simulink model "TinBotEliminator"  (Simulink 8.7)
settings: Solver=VariableStepAuto  StartTime=0.0  StopTime=10.0  RelTol=1e-3
settings Model: Creator=maximilian  LastModifiedBy=maximilian
settings DataIOCC: LimitDataPoints=off  SaveFormat=Dataset
settings DebuggingCC: UnderspecifiedInitializationDetection=Simplified  MergeDetectMultiDrivingBlocksExec=error
settings HardwareCC: ProdBitPerPointer=64  ProdLargestAtomicFloat=Float  ProdIntDivRoundTo=Zero  ProdEndianess=LittleEndian  ProdWordSize=64  ProdHWDeviceType=Intel->x86-64 (Windows64)
settings ModelReferenceCC: PropagateSignalLabelsOutOfModel=on
settings ConfigComp: CovModelRefEnable=off

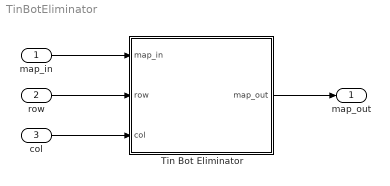
== system TinBotEliminator ==
  map_in : Inport  PortDimensions=[100 100]
  row : Inport  Port=2
  col : Inport  Port=3
  Tin Bot Eliminator : MATLAB Function  TreatAsAtomicUnit=on
  map_out : Outport  PortDimensions=[100 100]
  wires:
  map_in/1 -> Tin Bot Eliminator/1(map_in)
  row/1 -> Tin Bot Eliminator/2(row)
  col/1 -> Tin Bot Eliminator/3(col)
  Tin Bot Eliminator/1(map_out) -> map_out/1

== matlab function Tin Bot Eliminator ==
  data: map_in input double; map_out output double; row input double; col input double
function map_out = eliminate(map_in, row, col)
    map_in(row, col) = 0;
    map_out = map_in;
